simulink subsystem "IR_LEDs"  (R2024a)
settings: Solver=VariableStepAuto  StartTime=0.0  StopTime=10.0  RelTol=1e-3
libraries: stm32f4xxblockslib x8
settings Model: Creator=JesseJabezArendse  LastModifiedBy=masha
settings RTWCC: GPUComputeCapability=3.5

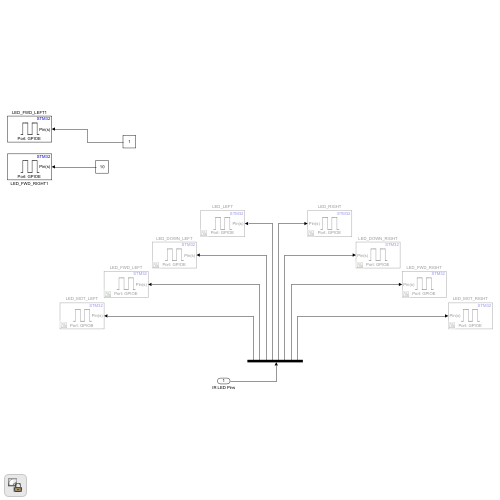
[thumbnail: Simulink's stored preview of the top-level diagram]
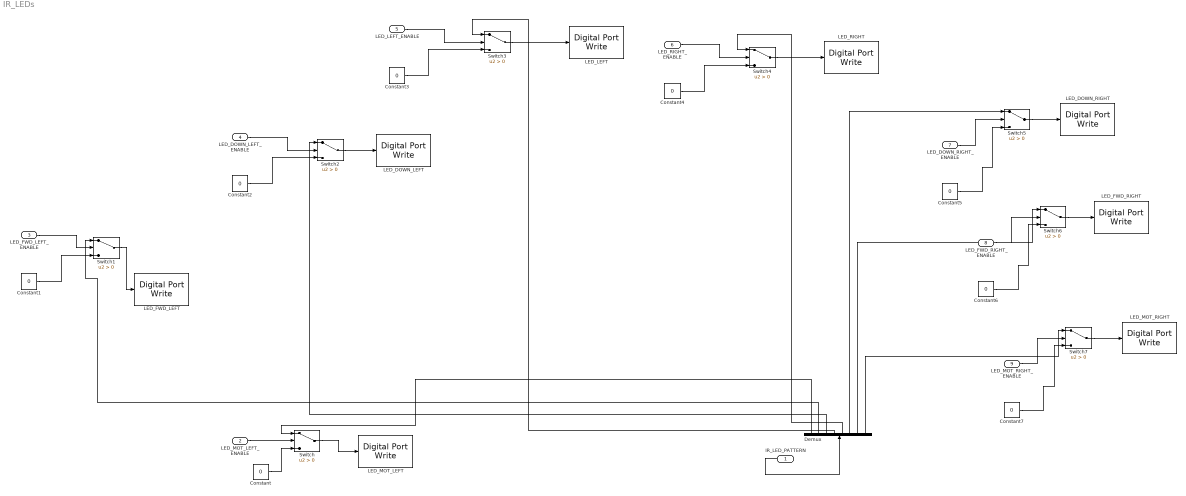
== system IR_LEDs ==
  IR_LED_PATTERN : Inport
  LED_MOT_LEFT_ENABLE : Inport  Port=2
  LED_FWD_LEFT_ENABLE : Inport  Port=3
  LED_DOWN_LEFT_ENABLE : Inport  Port=4
  LED_LEFT_ENABLE : Inport  Port=5
  LED_RIGHT_ENABLE : Inport  Port=6
  LED_DOWN_RIGHT_ENABLE : Inport  Port=7
  LED_FWD_RIGHT_ENABLE : Inport  Port=8
  LED_MOT_RIGHT_ENABLE : Inport  Port=9
  Constant{,1..7} (8 alike) : Constant  Value=0
  Demux : Demux  Outputs=8
  LED_DOWN_LEFT : stm32f4xxblockslib/Digital Port Write  PortName=GPIOE  PinNumber=9  ReadOperation=off  IOAsArray=on  EnableSimPort=off  hoistedMaskSrc=ECSoC/ECSimCodegen/Digital Port Write
      settings: LibrarySourceBlock=stm32l4xxblockslib/Digital Port Write
  LED_DOWN_RIGHT : stm32f4xxblockslib/Digital Port Write  PortName=GPIOE  PinNumber=14  ReadOperation=off  IOAsArray=on  EnableSimPort=off  hoistedMaskSrc=ECSoC/ECSimCodegen/Digital Port Write
      settings: LibrarySourceBlock=stm32l4xxblockslib/Digital Port Write
  LED_FWD_LEFT : stm32f4xxblockslib/Digital Port Write  PortName=GPIOE  PinNumber=8  ReadOperation=off  IOAsArray=on  EnableSimPort=off  hoistedMaskSrc=ECSoC/ECSimCodegen/Digital Port Write
      settings: LibrarySourceBlock=stm32l4xxblockslib/Digital Port Write
  LED_FWD_RIGHT : stm32f4xxblockslib/Digital Port Write  PortName=GPIOE  PinNumber=15  ReadOperation=off  IOAsArray=on  EnableSimPort=off  hoistedMaskSrc=ECSoC/ECSimCodegen/Digital Port Write
      settings: LibrarySourceBlock=stm32l4xxblockslib/Digital Port Write
  LED_LEFT : stm32f4xxblockslib/Digital Port Write  PortName=GPIOE  PinNumber=12  ReadOperation=off  IOAsArray=on  EnableSimPort=off  hoistedMaskSrc=ECSoC/ECSimCodegen/Digital Port Write
      settings: LibrarySourceBlock=stm32l4xxblockslib/Digital Port Write
  LED_MOT_LEFT : stm32f4xxblockslib/Digital Port Write  PortName=GPIOB  PinNumber=12  ReadOperation=off  IOAsArray=on  EnableSimPort=off  hoistedMaskSrc=ECSoC/ECSimCodegen/Digital Port Write
      settings: LibrarySourceBlock=stm32l4xxblockslib/Digital Port Write
  LED_MOT_RIGHT : stm32f4xxblockslib/Digital Port Write  PortName=GPIOE  PinNumber=13  ReadOperation=off  IOAsArray=on  EnableSimPort=off  hoistedMaskSrc=ECSoC/ECSimCodegen/Digital Port Write
      settings: LibrarySourceBlock=stm32l4xxblockslib/Digital Port Write
  LED_RIGHT : stm32f4xxblockslib/Digital Port Write  PortName=GPIOE  PinNumber=11  ReadOperation=off  IOAsArray=on  EnableSimPort=off  hoistedMaskSrc=ECSoC/ECSimCodegen/Digital Port Write
      settings: LibrarySourceBlock=stm32l4xxblockslib/Digital Port Write
  Switch{,1..7} (8 alike) : Switch  Criteria=u2 > Threshold  SaturateOnIntegerOverflow=off  InputSameDT=off
  wires:
  Demux/1 -> Switch/1
  Demux/2 -> Switch1/1
  Demux/4 -> Switch3/1
  Demux/5 -> Switch4/1
  Demux/7 -> Switch6/1
  Demux/8 -> Switch7/1
  Demux/3 -> Switch2/1
  Demux/6 -> Switch5/1
  IR_LED_PATTERN/1 -> Demux/1
  LED_MOT_LEFT_ENABLE/1 -> Switch/2
  Switch/1 -> LED_MOT_LEFT/1
  Constant/1 -> Switch/3
  LED_FWD_LEFT_ENABLE/1 -> Switch1/2
  Switch1/1 -> LED_FWD_LEFT/1
  Constant1/1 -> Switch1/3
  LED_DOWN_LEFT_ENABLE/1 -> Switch2/2
  Switch2/1 -> LED_DOWN_LEFT/1
  Constant2/1 -> Switch2/3
  Constant3/1 -> Switch3/3
  LED_LEFT_ENABLE/1 -> Switch3/2
  Switch3/1 -> LED_LEFT/1
  Constant4/1 -> Switch4/3
  LED_RIGHT_ENABLE/1 -> Switch4/2
  Switch4/1 -> LED_RIGHT/1
  Constant5/1 -> Switch5/3
  LED_DOWN_RIGHT_ENABLE/1 -> Switch5/2
  Switch5/1 -> LED_DOWN_RIGHT/1
  Switch6/1 -> LED_FWD_RIGHT/1
  Constant6/1 -> Switch6/3
  LED_FWD_RIGHT_ENABLE/1 -> Switch6/2
  Switch7/1 -> LED_MOT_RIGHT/1
  Constant7/1 -> Switch7/3
  LED_MOT_RIGHT_ENABLE/1 -> Switch7/2
